simulink model "DAB_OL_2"  (R2023b)
settings: Solver=VariableStepAuto  StartTime=0.0  StopTime=5  RelTol=1e-3
undefined symbols (not defined in the file): Ion, Lithium
libraries: spsVoltageMeasurementLib x10, spsMosfetLib x8, spsSeriesRLCBranchLib x4, spsMeanLib x4, spsCurrentMeasurementLib x3, spsBatteryLib x1, spsDCVoltageSourceLib x1, spsLinearTransformerLib x1, spsRMSLib x1, spspowerguiLib x1
settings Model: SimulationMode=rapid-accelerator  Creator=Project_Account  LastModifiedBy=USER
settings ModelReferenceCC: EnableRefExpFcnMdlSchedulingChecks=on

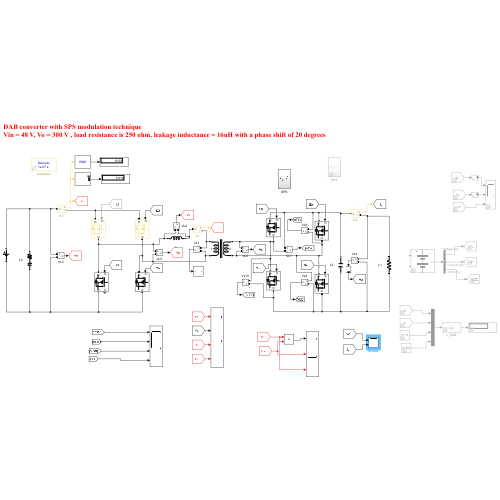
[thumbnail: Simulink's stored preview of the top-level diagram]
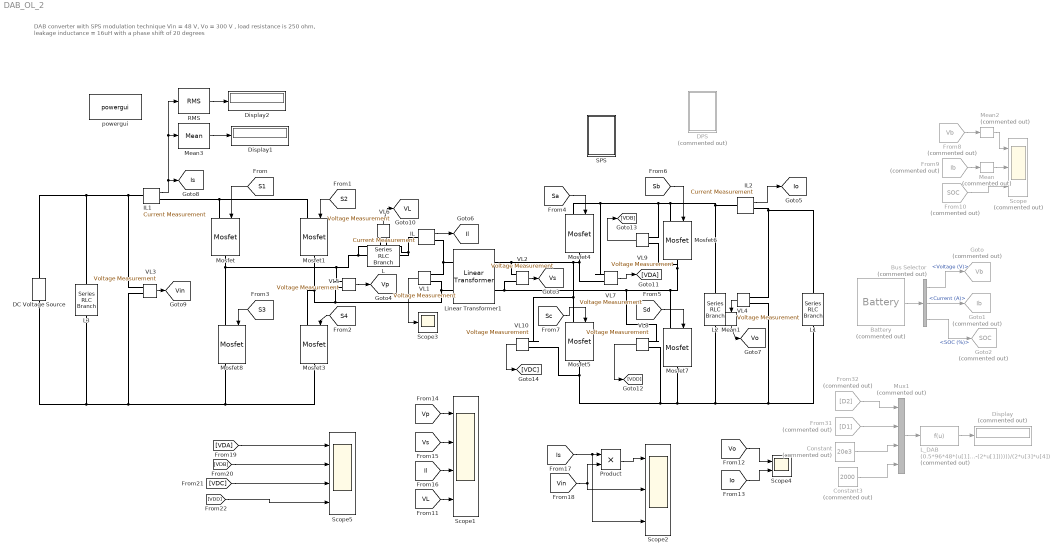
== system DAB_OL_2 ==
  note: DAB converter with SPS modulation technique
      | Vin = 48 V, Vo = 300 V , load resistance is 250 ohm, leakage inductance = 16uH with a phase shift of 20 degrees
  Battery : spsBatteryLib/Battery  Commented=on  BatType=Lithium-Ion  ShowTempParam=off  ThermalPreset=no  ShowAgeParam=off  NomV=48  NomQ=50  SOC=60  Batt_Tr=0.1  PresetModel=on  MaxQ=50  MinV=36  FullV=55.8714  Dis_rate=21.7391  R=0.0096  Normal_OP=45.2174  expZone="[51.8585      2.45652]"  current=[6.5 13 32.5]  Units=Time  Tci=20  NomT=20  T2=-30  MaxQ2=4.8  FullV2=7.1  Normal_OP2=5.655  expZone2="[6.58           1]"  Rca=0.6  ti=2000  Dp=0  Neq0=0  Tsim=1e6  Ta1=25  Qeol=5.4*0.9  Reol=0.013333*1.2  Char_age=[2.3478, 3]  Dis_age=[2.3478, 10]  N1=1500  N2=10500  N3=1000  N4=1400  Ta2=45  N5=950
  Bus Selector : BusSelector  Commented=on  OutputSignals=Voltage (V),Current (A),SOC (%)
  Constant : Constant  Commented=on  Value=20e3
  Constant3 : Constant  Commented=on  Value=2000
  DC Voltage Source : spsDCVoltageSourceLib/DC Voltage Source  Amplitude=48  Measurements=None
  DPS : Subsystem  Commented=on
  Display : Display  Commented=on
  Display1 : Display
  Display2 : Display
  From10 : From  Commented=on  GotoTag=SOC  TagVisibility=global
  From31 : From  Commented=on  GotoTag=D1  TagVisibility=global
  From32 : From  Commented=on  GotoTag=D2  TagVisibility=global
  From8 : From  Commented=on  GotoTag=Vb  TagVisibility=global
  From9 : From  Commented=on  GotoTag=Ib  TagVisibility=global
  Goto : Goto  Commented=on  GotoTag=Vb  TagVisibility=global
  Goto1 : Goto  Commented=on  GotoTag=Ib  TagVisibility=global
  Goto2 : Goto  Commented=on  GotoTag=SOC  TagVisibility=global
  IL : spsCurrentMeasurementLib/Current Measurement  PhasorSimulation=off  OutputType=Complex  PSBequivalent=0
  IL1 : spsCurrentMeasurementLib/Current Measurement  PhasorSimulation=off  OutputType=Complex  PSBequivalent=0
  IL2 : spsCurrentMeasurementLib/Current Measurement  PhasorSimulation=off  OutputType=Complex  PSBequivalent=0
  L : spsSeriesRLCBranchLib/Series RLC Branch  LConnTagsString=__new0  RConnTagsString=__new0  BranchType=L  Resistance=1  Inductance=16e-6  SetiL0=off  InitialCurrent=0  Capacitance=1e-6  Setx0=off  InitialVoltage=0  Measurements=None
  L1 : spsSeriesRLCBranchLib/Series RLC Branch  LConnTagsString=__new0  RConnTagsString=__new0  BranchType=R  Resistance=250  Inductance=19.108e-6*2  SetiL0=off  InitialCurrent=0  Capacitance=1000e-6  Setx0=off  InitialVoltage=0  Measurements=None
  L2 : spsSeriesRLCBranchLib/Series RLC Branch  LConnTagsString=__new0  RConnTagsString=__new0  BranchType=C  Resistance=0.8  Inductance=19.108e-6*2  SetiL0=off  InitialCurrent=0  Capacitance=1200e-6  Setx0=off  InitialVoltage=0  Measurements=None
  L3 : spsSeriesRLCBranchLib/Series RLC Branch  LConnTagsString=__new0  RConnTagsString=__new0  BranchType=RC  Resistance=0.8  Inductance=19.108e-6*2  SetiL0=off  InitialCurrent=0  Capacitance=1200e-6  Setx0=off  InitialVoltage=0  Measurements=None
  L_DAB : Fcn  Commented=on  Expr=(0.5*96*48*(u[1]*(1-u[1])+((u[2]/2)*(1-u[2]-(2*u[1])))))/(2*u[3]*u[4])
  Linear Transformer1 : spsLinearTransformerLib/Linear Transformer  UNITS=SI  NominalPower=[1500 15000 ]  winding1=[48 0 0]  winding2=[300 0 0]  ThreeWindings=off  winding3=[3.15e+05 0.7938 0.084225]  RmLm=[5000 5866]  Measurements=None  DataType=on
  Mean : spsMeanLib/Mean  Commented=on  Freq=20000  Vinit=0  Ts=1e-7
  Mean1 : spsMeanLib/Mean  Freq=20000  Vinit=0  Ts=1e-7
  Mean2 : spsMeanLib/Mean  Commented=on  Freq=20000  Vinit=0  Ts=1e-7
  Mean3 : spsMeanLib/Mean  Freq=15000  Vinit=0  Ts=1e-6
  Mosfet{,1,3..7} (7 alike) : spsMosfetLib/Mosfet  Ron=0.1  Lon=0  Rd=0.01  Vfd=0  IC=0  Rs=1e5  Cs=inf  Measurements=off
  Mosfet8 : spsMosfetLib/Mosfet  Ron=0.1  Lon=0  Rd=0.01  Vfd=0  IC=0  Rs=1e5  Cs=inf  Measurements=on
  Mux1 : Mux  Commented=on
  Product : Product
  RMS : spsRMSLib/RMS  TrueRMS=on  Freq=60  RMSInit=120  Ts=0
  SPS : Subsystem
  Scope : Scope  Commented=on  NumInputPorts=3
  Scope1 : Scope  NumInputPorts=4
  Scope2 : Scope  NumInputPorts=3
  Scope3 : Scope
  Scope4 : Scope  NumInputPorts=2
  Scope5 : Scope  NumInputPorts=4
  VL{1..10} (10 alike) : spsVoltageMeasurementLib/Voltage Measurement  PhasorSimulation=off  OutputType=Complex  PSBequivalent=0
  powergui : spspowerguiLib/powergui  Priority=1  SimulationMode=Discrete  SampleTime=1e-7  frequency=60  Iterations=50  frequencyindice=0  Pbase=100e6  ErrMax=1e-4  UnitsV=kV  UnitsW=MW  buscounter=0  FunctionMessages=off  echomessages=off  EnableUseOfTLC=off  CurrentSourceSwitches=off  DisableSnubberDevices=off  DisableRonSwitches=off  DisableVfSwitches=off  DisplayEquations=off  AutomaticDiscreteSolvers=off  SolverType=Tustin/Backward Euler (TBE)  Interpol=off  ExternalGateDelay=off  methode=off  Ts=100  x0status=blocks  SPID=on  SwTol=0  HookPort=off  NonlinearTolerance=1e-6  nMaxIteration=1000  ContinueOnMaxIteration=off  RestoreLinks=warning  ResistiveCurrentMeasurement=off  Frange=[0:2:500]  Ylog=off  Xlog=on  ShowGrid=off  save=off  variable=ZData  structure=0  ZoomFFT=off  StartTime=0.0  cycles=1  DisplayStyle=1  fundamental=60  FreqAxis=off  MaxFrequency=1000  frequencyindicesteady=1  RmsSteady=1  display=off
  tag scope: Il=global, Io=global, Is=global, VL=global, Vin=global, Vo=global, Vp=global, Vs=global
  wires:
  VL1/1 -> Scope3/1
  [Il] -> Scope1/3
  [S3] -> Mosfet8/1
  Mean2/1 -> Scope/1
  [Sb] -> Mosfet6/1
  From9/1 -> Mean/1
  From8/1 -> Mean2/1
  [Sc] -> Mosfet5/1
  From31/1 -> Mux1/2
  Mean1/1 -> [Vo]
  [Vin] -> Scope2/2, Product/2
  [Vo] -> Scope4/1
  VL6/1 -> [VL]
  IL2/1 -> [Io]
  [S2] -> Mosfet1/1
  VL3/1 -> [Vin]
  [S4] -> Mosfet3/1
  [Is] -> Scope2/3, Product/1
  Product/1 -> Scope2/1
  VL5/1 -> [Vp]
  Mean3/1 -> Display1/1
  IL1/1 -> RMS/1, Mean3/1, [Is]
  Bus Selector/1 -> Goto/1  "<Voltage (V)>"
  [Sd] -> Mosfet7/1
  L_DAB/1 -> Display/1
  RMS/1 -> Display2/1
  [Io] -> Scope4/2
  VL2/1 -> [Vs]
  Constant/1 -> Mux1/3
  Mean/1 -> Scope/2
  From10/1 -> Scope/3
  Mux1/1 -> L_DAB/1
  VL4/1 -> Mean1/1
  [S1] -> Mosfet/1
  [Vp] -> Scope1/1
  Bus Selector/2 -> Goto1/1  "<Current (A)>"
  IL/1 -> [Il]
  [Sa] -> Mosfet4/1
  [Vs] -> Scope1/2
  Constant3/1 -> Mux1/4
  From32/1 -> Mux1/1
  Battery/1 -> Bus Selector/1
  Bus Selector/3 -> Goto2/1  "<SOC (%)>"
  [VL] -> Scope1/4
  VL7/1 -> [VDA]
  [VDA] -> Scope5/1
  VL8/1 -> [VDD]
  [VDD] -> Scope5/4
  VL9/1 -> [VDB]
  VL10/1 -> [VDC]
  [VDB] -> Scope5/2
  [VDC] -> Scope5/3
  connections:
  Mosfet7/LConn1 -- VL2/LConn2 -- Linear Transformer1/RConn2 -- VL8/LConn2 -- VL9/LConn1 -- Mosfet6/RConn1
  IL/LConn1 -- VL6/LConn2 -- L/RConn1
  Linear Transformer1/RConn1 -- Mosfet5/LConn1 -- VL10/LConn2 -- VL7/LConn2 -- Mosfet4/RConn1 -- VL2/LConn1
  VL5/LConn2 -- VL1/LConn2 -- Linear Transformer1/LConn2 -- Mosfet3/LConn1 -- Mosfet1/RConn1
  VL1/LConn1 -- IL/RConn1 -- Linear Transformer1/LConn1
  Mosfet3/RConn1 -- Mosfet8/RConn1 -- DC Voltage Source/LConn1 -- L3/RConn1 -- VL3/LConn2
  VL5/LConn1 -- Mosfet/RConn1 -- Mosfet8/LConn1 -- L/LConn1 -- VL6/LConn1
  VL3/LConn1 -- IL1/LConn1 -- L3/LConn1 -- DC Voltage Source/RConn1
  Mosfet/LConn1 -- IL1/RConn1 -- Mosfet1/LConn1
  L1/LConn1 -- VL4/LConn1 -- IL2/RConn1
  Mosfet4/LConn1 -- VL7/LConn1 -- VL9/LConn2 -- Mosfet6/LConn1 -- L2/LConn1 -- IL2/LConn1
  L1/RConn1 -- L2/RConn1 -- VL10/LConn1 -- Mosfet5/RConn1 -- VL8/LConn1 -- Mosfet7/RConn1 -- VL4/LConn2

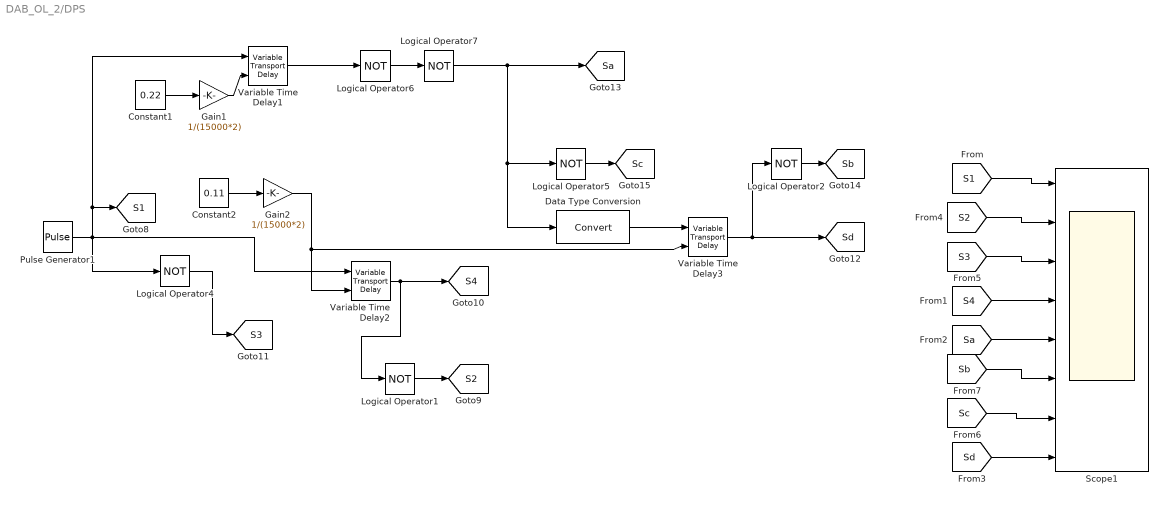
== system DAB_OL_2/DPS ==
  Constant1 : Constant  Value=0.22
  Constant2 : Constant  Value=0.11
  Data Type Conversion : DataTypeConversion  SaturateOnIntegerOverflow=off  RndMeth=Floor
  Gain1 : Gain  Gain=1/(15000*2)
  Gain2 : Gain  Gain=1/(15000*2)
  Logical Operator{1..2,4..7} (6 alike) : Logic  Operator=NOT  AllPortsSameDT=off  OutDataTypeStr=boolean
  Pulse Generator1 : DiscretePulseGenerator  PulseType=Time based  Period=1/(15000*2)  PulseWidth=50
  Scope1 : Scope  NumInputPorts=8
  Variable Time Delay1 : VariableTransportDelay  MaximumDelay=10
  Variable Time Delay2 : VariableTransportDelay  MaximumDelay=10
  Variable Time Delay3 : VariableTransportDelay  MaximumDelay=10
  tag scope: S1=global, S2=global, S3=global, S4=global, Sa=global, Sb=global, Sc=global, Sd=global
  wires:
  Constant1/1 -> Gain1/1
  Gain1/1 -> Variable Time Delay1/2
  Variable Time Delay1/1 -> Logical Operator6/1
  Variable Time Delay3/1 -> Logical Operator2/1, [Sd]
  Logical Operator6/1 -> Logical Operator7/1
  Pulse Generator1/1 -> Variable Time Delay2/1, Variable Time Delay1/1, [S1], Logical Operator4/1
  Logical Operator7/1 -> [Sa], Logical Operator5/1, Data Type Conversion/1
  Constant2/1 -> Gain2/1
  Gain2/1 -> Variable Time Delay3/2, Variable Time Delay2/2
  Variable Time Delay2/1 -> Logical Operator1/1, [S4]
  Logical Operator1/1 -> [S2]
  Logical Operator4/1 -> [S3]
  Logical Operator5/1 -> [Sc]
  Logical Operator2/1 -> [Sb]
  Data Type Conversion/1 -> Variable Time Delay3/1
  [S1] -> Scope1/1
  [Sa] -> Scope1/5
  [S4] -> Scope1/4
  [S2] -> Scope1/2
  [S3] -> Scope1/3
  [Sd] -> Scope1/8
  [Sc] -> Scope1/7
  [Sb] -> Scope1/6

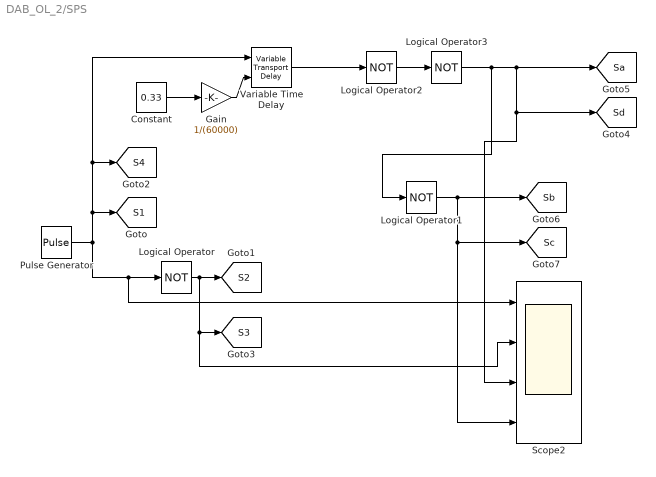
== system DAB_OL_2/SPS ==
  Constant : Constant  Value=0.33
  Gain : Gain  Gain=1/(60000)
  Logical Operator{,1..3} (4 alike) : Logic  Operator=NOT  AllPortsSameDT=off  OutDataTypeStr=boolean
  Pulse Generator : DiscretePulseGenerator  PulseType=Time based  Period=1/(60000)  PulseWidth=50
  Scope2 : Scope  NumInputPorts=4
  Variable Time Delay : VariableTransportDelay  MaximumDelay=10
  tag scope: S1=global, S2=global, S3=global, S4=global, Sa=global, Sb=global, Sc=global, Sd=global
  wires:
  Logical Operator2/1 -> Logical Operator3/1
  Logical Operator3/1 -> Logical Operator1/1, [Sa], Scope2/3, [Sd]
  Logical Operator1/1 -> Scope2/4, [Sc], [Sb]
  Pulse Generator/1 -> Variable Time Delay/1, [S4], [S1], Scope2/1, Logical Operator/1
  Logical Operator/1 -> Scope2/2, [S3], [S2]
  Gain/1 -> Variable Time Delay/2
  Variable Time Delay/1 -> Logical Operator2/1
  Constant/1 -> Gain/1
